simulink subsystem "RT_RelativeWindOnAllBlade"  (R2025a)
settings: Solver=VariableStepAuto  StartTime=0.0  StopTime=10  RelTol=1e-3
undefined symbols (not defined in the file): RT_BEDistFromEffSta_A, RT_BladeSegment_P, RT_HubOffsetBody_P, RT_ShaftTiltFwd_P, RT_ShaftTiltRight_P
settings Model: DataDictionary=Rotor.sldd  EnableAccessToBaseWorkspace=off  DefaultTestHarness=RT_RelativeWindOnAllBlade_Harness  Creator=tunglt60  LastModifiedBy=tunglt60

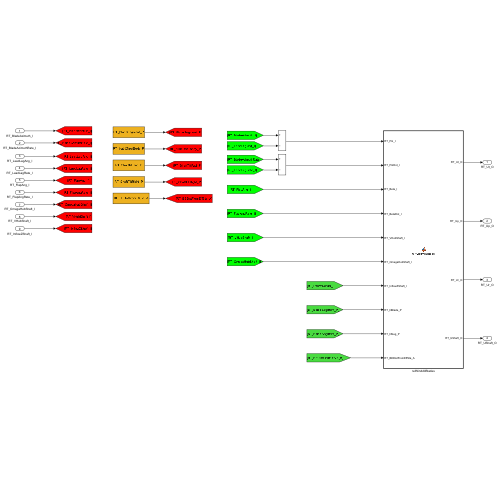
[thumbnail: Simulink's stored preview of the top-level diagram]
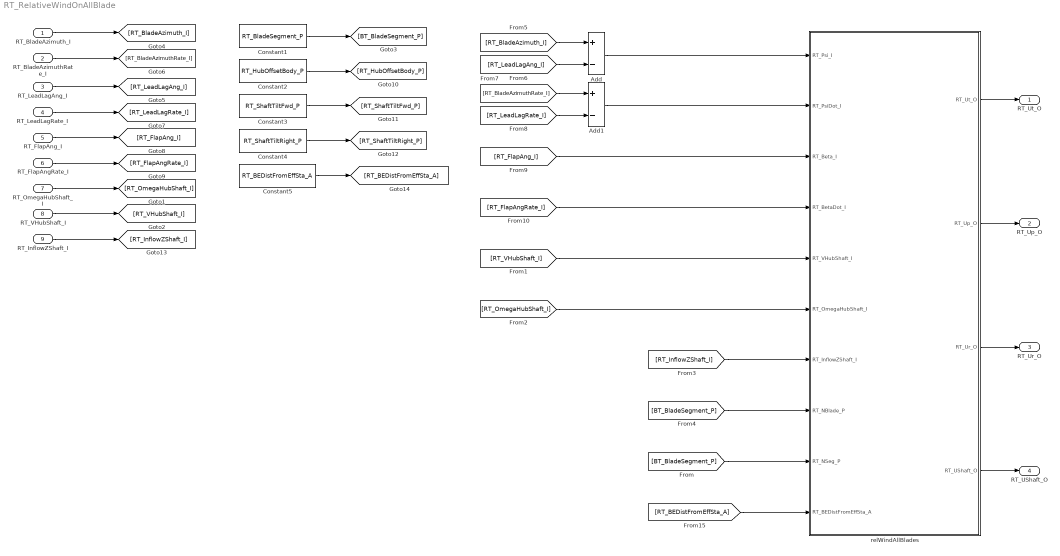
== system RT_RelativeWindOnAllBlade ==
  RT_BladeAzimuth_I : Inport
  RT_BladeAzimuthRate_I : Inport  Port=2
  RT_LeadLagAng_I : Inport  Port=3
  RT_LeadLagRate_I : Inport  Port=4
  RT_FlapAng_I : Inport  Port=5
  RT_FlapAngRate_I : Inport  Port=6
  RT_OmegaHubShaft_I : Inport  Port=7
  RT_VHubShaft_I : Inport  Port=8
  RT_InflowZShaft_I : Inport  Port=9
  Add : Sum  Inputs=+-
  Add1 : Sum  Inputs=+-
  Constant1 : Constant  Value=RT_BladeSegment_P
  Constant2 : Constant  Value=RT_HubOffsetBody_P
  Constant3 : Constant  Value=RT_ShaftTiltFwd_P
  Constant4 : Constant  Value=RT_ShaftTiltRight_P
  Constant5 : Constant  Value=RT_BEDistFromEffSta_A
  relWindAllBlades : MATLAB Function  TreatAsAtomicUnit=on
  RT_Ut_O : Outport
  RT_Up_O : Outport  Port=2
  RT_Ur_O : Outport  Port=3
  RT_UShaft_O : Outport  Port=4
  wires:
  [RT_LeadLagAng_I] -> Add/2
  RT_FlapAng_I/1 -> [RT_FlapAng_I]
  RT_BladeAzimuthRate_I/1 -> [RT_BladeAzimuthRate_I]
  RT_FlapAngRate_I/1 -> [RT_FlapAngRate_I]
  RT_LeadLagRate_I/1 -> [RT_LeadLagRate_I]
  RT_BladeAzimuth_I/1 -> [RT_BladeAzimuth_I]
  Constant1/1 -> [BT_BladeSegment_P]
  relWindAllBlades/3(RT_Ur_O) -> RT_Ur_O/1
  Constant5/1 -> [RT_BEDistFromEffSta_A]
  relWindAllBlades/1(RT_Ut_O) -> RT_Ut_O/1
  relWindAllBlades/4(RT_UShaft_O) -> RT_UShaft_O/1
  RT_InflowZShaft_I/1 -> [RT_InflowZShaft_I]
  RT_VHubShaft_I/1 -> [RT_VHubShaft_I]
  relWindAllBlades/2(RT_Up_O) -> RT_Up_O/1
  [BT_BladeSegment_P] -> relWindAllBlades/9(RT_NSeg_P)
  RT_LeadLagAng_I/1 -> [RT_LeadLagAng_I]
  [RT_InflowZShaft_I] -> relWindAllBlades/7(RT_InflowZShaft_I)
  RT_OmegaHubShaft_I/1 -> [RT_OmegaHubShaft_I]
  Constant2/1 -> [RT_HubOffsetBody_P]
  [RT_LeadLagRate_I] -> Add1/2
  Constant3/1 -> [RT_ShaftTiltFwd_P]
  Constant4/1 -> [RT_ShaftTiltRight_P]
  [RT_BladeAzimuth_I] -> Add/1
  Add1/1 -> relWindAllBlades/2(RT_PsiDot_I)
  Add/1 -> relWindAllBlades/1(RT_Psi_I)
  [RT_VHubShaft_I] -> relWindAllBlades/5(RT_VHubShaft_I)
  [RT_FlapAng_I] -> relWindAllBlades/3(RT_Beta_I)
  [RT_BladeAzimuthRate_I] -> Add1/1
  [RT_BEDistFromEffSta_A] -> relWindAllBlades/10(RT_BEDistFromEffSta_A)
  [RT_FlapAngRate_I] -> relWindAllBlades/4(RT_BetaDot_I)
  [BT_BladeSegment_P] -> relWindAllBlades/8(RT_NBlade_P)
  [RT_OmegaHubShaft_I] -> relWindAllBlades/6(RT_OmegaHubShaft_I)

== matlab function RT_RelativeWindOnAllBlade/relWindAllBlades ==
  data: RT_Psi_I input; RT_Ut_O output; RT_PsiDot_I input; RT_Beta_I input; RT_BetaDot_I input; RT_VHubShaft_I input; RT_OmegaHubShaft_I input; RT_InflowZShaft_I input; RT_NBlade_P input; RT_NSeg_P input; RT_Up_O output; RT_Ur_O output; RT_UShaft_O output; RT_BEDistFromEffSta_A input
function [RT_Ut_O, RT_Up_O, RT_Ur_O, RT_UShaft_O] = ...
    relWindAllBlades( ...
        RT_Psi_I, RT_PsiDot_I, RT_Beta_I, RT_BetaDot_I, ...
        RT_VHubShaft_I, RT_OmegaHubShaft_I, RT_InflowZShaft_I, ...
        RT_NBlade_P, RT_NSeg_P, RT_BEDistFromEffSta_A)
%RELWINDALLBLADES  Relative wind for every blade/element of a rotor.
%
%   All vectors in SHAFT frame. Hub kinematics (VHubShaft, OmegaHubShaft)
%   are expressed RELATIVE TO THE AMBIENT AIR MASS -- i.e. the caller has
%   already subtracted wind velocity from the earth-frame hub velocity.
%
%   Because of that, the only non-zero component of the air velocity at
%   each blade element is the rotor-INDUCED INFLOW along shaft +z. The
%   function therefore takes inflow as a SCALAR per (blade, element)
%   instead of a full 3-vector field.
%
%   Sign conventions
%   ----------------
%     shaft +z points DOWN
%     beta > 0 : flap up
%     UT > 0   : tangential, opposite to rotation (+eT = -sign(dpsi)*eA)
%     UP > 0   : perpendicular to chord plane (+eP); = +z only at beta=0
%     UR > 0   : radial, root -> tip (+eR)
%     inflow z > 0 : air pushed DOWN through the disk
%
%   Inputs
%   ------
%     RT_Psi_I               [NB x NSeg]   azimuth                      [rad]
%     RT_PsiDot_I            [NB x NSeg]   azimuth rate                 [rad/s]
%     RT_Beta_I              [NB x NSeg]   flap angle                   [rad]
%     RT_BetaDot_I           [NB x NSeg]   flap rate                    [rad/s]
%     RT_VHubShaft_I         [3 x 1]       hub velocity vs air mass     [m/s]
%     RT_OmegaHubShaft_I     [3 x 1]       hub angular rate             [rad/s]
%     RT_InflowZShaft_I      [NB x NSeg]   induced inflow, +z down      [m/s]
%     RT_NBlade_P            scalar        number of blades NB
%     RT_NSeg_P              scalar        elements per blade
%     RT_BEDistFromEffSta_A  [1 x NSeg]    element station radii        [m]
%
%   Outputs
%   -------
%     RT_Ut_O                [NB x NSeg]       tangential             [m/s]
%     RT_Up_O                [NB x NSeg]       perpendicular to chord [m/s]
%     RT_Ur_O                [NB x NSeg]       radial                 [m/s]
%     RT_UShaft_O            [3 x NSeg x NB]   relative wind vector   [m/s]
%
% ------------------------------------------------------------------------

    % ----- 0. Preallocation ----------------------------------------------
    nB   = RT_NBlade_P;
    nSeg = RT_NSeg_P;
    [nB, nSeg] = size(RT_Psi_I);

    RT_Ut_O        = zeros(nB, nSeg);
    RT_Up_O        = zeros(nB, nSeg);
    RT_Ur_O        = zeros(nB, nSeg);
    RT_UShaft_O    = zeros(3, nSeg, nB);

    ez = [0; 0; 1];   % +z_shaft is DOWN

    % Hub kinematics shared by all blades / elements (air-mass frame).
    vHub  = RT_VHubShaft_I(:);
    omHub = RT_OmegaHubShaft_I(:);

    % ----- 1. Double loop: blade -> element ------------------------------
    for b = 1:nB
        for k = 1:nSeg

            % --- 1.1 Scalars for this element ---------------------------
            rk     = RT_BEDistFromEffSta_A(k);
            psi    = RT_Psi_I(b, k);
            dpsi   = RT_PsiDot_I(b, k);
            beta   = RT_Beta_I(b, k);
            dbeta  = RT_BetaDot_I(b, k);
            inflow = RT_InflowZShaft_I(b, k);     % scalar, +z component



            cp = cos(psi);  sp = sin(psi);
            cb = cos(beta); sb = sin(beta);

            % --- 1.2 Element frame (eR, eA, eP, eT) ---------------------
            % eR0 : radial in hub plane (no flap), from hub outward
            % eA  : azimuthal, in hub plane, along +dpsi direction
            %       (eR0 x eA = ez, so (eR0, eA, ez) is right-handed)
            % eR  : radial with flap = cos(beta)*eR0 - sin(beta)*ez
            %       (the -sb*ez term tilts the tip upward since +z is DOWN)
            % eP  : normal to the blade chord plane = eR x eA
            %       (reduces to ez when beta = 0; tilts with the blade otherwise)
            % eT  : tangential, opposite to the rotation sense = -sign(dpsi)*eA
            eR0 = [-cp;  sp; 0.0];
            eA  = [sp;  cp; 0.0];
            eR  = cb * eR0 - sb * ez;
            eP  = cross(eA, eR);

            if dpsi == 0
                sgn = 1;
            else
                sgn = sign(dpsi);
            end
            eT = -sgn * eA;

            % --- 1.3 Position & velocity relative to hub ----------------
            % rSeg = rk * eR                         (position in shaft frame)
            %
            % vRel = d(rk * eR)/dt = rk * d(eR)/dt
            %      = rk * cos(beta) * dpsi * eA      <- rotation part
            %        - rk * dbeta * eP               <- flap part
            %   (because d(eR)/dt = cos(beta)*dpsi*eA - dbeta*eP)
            rSeg = rk * eR;
            vRel = rk * cb * dpsi * eA - rk * dbeta * eP;

            % --- 1.4 Absolute velocity of the element in shaft frame ----
            % vSeg = vHub + omHub x rSeg + vRel
            %        (vHub already in air-mass frame, so vSeg is too)
            vSeg = vHub + cross(omHub, rSeg) + vRel;

            % --- 1.5 Relative wind = air - structure --------------------
            % Air velocity at this element is just [0; 0; inflow] in the
            % shaft frame (air-mass frame has no freestream component).
            %   u = [0; 0; inflow] - vSeg
            %     = [-vSeg(1); -vSeg(2); inflow - vSeg(3)]
            uX = -vSeg(1);
            uY = -vSeg(2);
            uZ = inflow - vSeg(3);
            RT_UShaft_O(:, k, b) = [uX; uY; uZ];

            % --- 1.6 Project onto (eT, eP, eR) --------------------------
            % For any unit vector e:
            %   dot([0;0;inflow] - vSeg, e)
            %     = inflow * e(3) - dot(vSeg, e)
            % This avoids materialising the air-velocity 3-vector and
            % saves one add per projection.
            RT_Ut_O(b, k) = inflow * eT(3) - (vSeg(1)*eT(1) + vSeg(2)*eT(2) + vSeg(3)*eT(3));
            RT_Up_O(b, k) = inflow * eP(3) - (vSeg(1)*eP(1) + vSeg(2)*eP(2) + vSeg(3)*eP(3));
            RT_Ur_O(b, k) = inflow * eR(3) - (vSeg(1)*eR(1) + vSeg(2)*eR(2) + vSeg(3)*eR(3));
        end
    end
end
